simulink model "SimulArm_Sliders"  (R2025b)
settings: Solver=VariableStepAuto  StartTime=0.0  StopTime=100  RelTol=1e-3  AbsTol=1e-3  EnableMultiTasking=on
values from neighbouring files (symbols this model uses):
  C = U * V'    [DataCondition.m]
  g = 9.80665    [DataCondition.m]
  N = numel(raw)    [DataCondition.m]
undefined symbols (not defined in the file or in its folder): X, Y, Z
libraries: sm_lib x45, nesl_utility x24, aerolibconvert2 x5, simulink x1
(part 1 of 3)
settings Model: SimulationMode=accelerator  Creator=ricky  LastModifiedBy=ricky
settings SolverCC: AutoScaleAbsTol=off  AlgebraicLoopSolver=TrustRegion  MaxZcPerStep=1.0
settings DataIOCC: LimitDataPoints=on  MaxDataPoints=10000
settings OptimizationCC: ReuseModelBlockBuffer=off  LifeSpan=inf
settings DebuggingCC: UnconnectedInputMsg=warning  UnconnectedOutputMsg=warning  UnconnectedLineMsg=warning  AllowSymbolicDim=off  SubsystemReferenceDiagnosticForUnitTest=warning  SFUnexpectedBacktrackingDiag=warning  SFNoUnconditionalDefaultTransitionDiag=warning  SFExecutionAtInitializationDiag=none  ArithmeticOperatorsInVariantConditions=warning
settings ModelReferenceCC: EnableRefExpFcnMdlSchedulingChecks=on
settings SFSimCC: SimUseLocalCustomCode=off  CustomCodeUndefinedFunction=UseInterfaceOnly
settings RTWCC: RTWUseLocalCustomCode=off  GPUComputeCapability=3.5  DLArmComputeVersion=19.05
settings CodeAppCC: StateflowObjectComments=on
settings GRTTargetCC: TargetLangStandard=C89/C90 (ANSI)
settings ConfigComp: CovMetricSettings=dw  CovSaveCumulativeToWorkspaceVar=on  CovSaveSingleToWorkspaceVar=on  CovExternalEMLEnable=off  CovSFcnEnable=off
settings SimscapeCC: SimscapeLogType=all  SimscapeLogSimulationStatistics=on  SimscapeLogDataHistory=10000.0

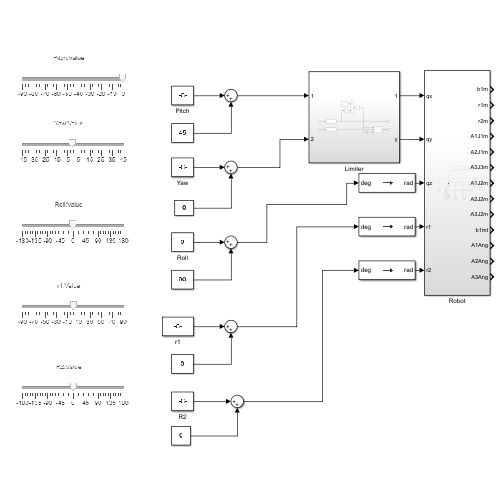
[thumbnail: Simulink's stored preview of the top-level diagram]
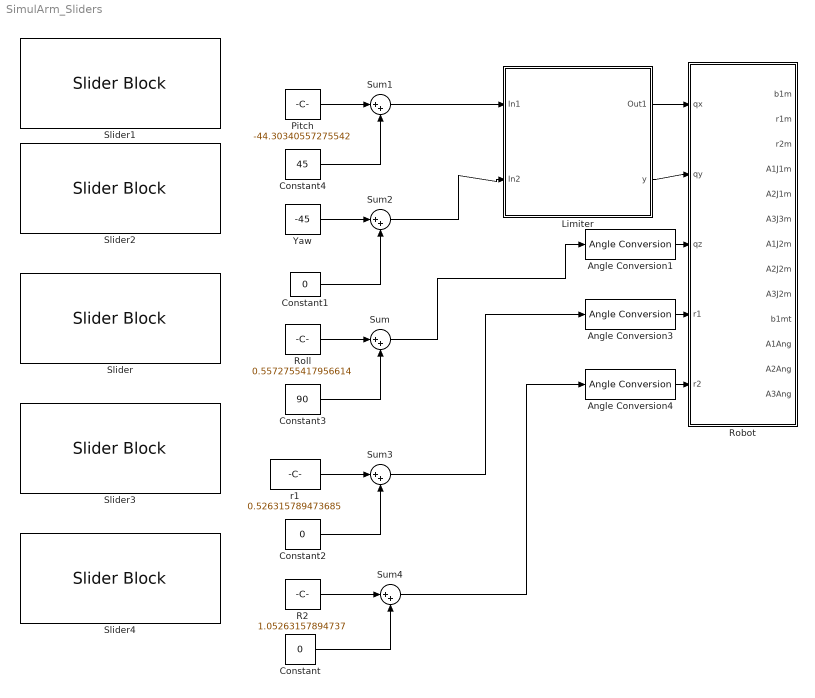
== system SimulArm_Sliders ==
  Angle Conversion1 : aerolibconvert2/Angle Conversion  IU=deg  OU=rad
  Angle Conversion3 : aerolibconvert2/Angle Conversion  IU=deg  OU=rad
  Angle Conversion4 : aerolibconvert2/Angle Conversion  IU=deg  OU=rad
  Constant : Constant  Value=0
  Constant1 : Constant  Value=0
  Constant2 : Constant  Value=0
  Constant3 : Constant  Value=90
  Constant4 : Constant  Value=45
  Limiter : Subsystem
  Pitch : Constant  Value=-44.30340557275542
  R2 : Constant  Value=1.05263157894737
  Robot : Subsystem
  Roll : Constant  Value=0.5572755417956614
  Slider : SliderBlock  ScaleMin=-180  ScaleMax=180
  Slider1 : SliderBlock  ScaleMin=-90  ScaleMax=0
  Slider2 : SliderBlock  ScaleMin=-45  ScaleMax=45
  Slider3 : SliderBlock  ScaleMin=-90  ScaleMax=90
  Slider4 : SliderBlock  ScaleMin=-180  ScaleMax=180
  Sum{,1..4} (5 alike) : Sum  Inputs=|++
  Yaw : Constant  Value=-45
  r1 : Constant  Value=0.526315789473685
  wires:
  Angle Conversion1/1 -> Robot/3(qz)
  Sum/1 -> Angle Conversion1/1
  Constant3/1 -> Sum/2
  Constant4/1 -> Sum1/2
  Constant1/1 -> Sum2/2
  Roll/1 -> Sum/1
  Angle Conversion3/1 -> Robot/4(r1)
  Angle Conversion4/1 -> Robot/5(r2)
  r1/1 -> Sum3/1
  Constant2/1 -> Sum3/2
  R2/1 -> Sum4/1
  Constant/1 -> Sum4/2
  Sum3/1 -> Angle Conversion3/1
  Sum4/1 -> Angle Conversion4/1
  Pitch/1 -> Sum1/1
  Yaw/1 -> Sum2/1
  Sum1/1 -> Limiter/1(In1)
  Sum2/1 -> Limiter/2(In2)
  Limiter/1(Out1) -> Robot/1(qx)
  Limiter/2(y) -> Robot/2(qy)

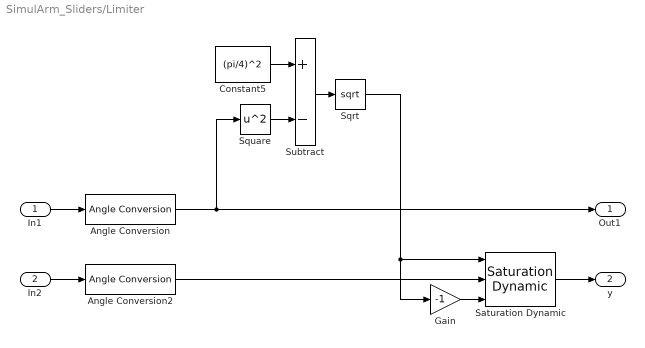
== system SimulArm_Sliders/Limiter ==
  In1 : Inport
  In2 : Inport  Port=2
  Angle Conversion : aerolibconvert2/Angle Conversion  IU=deg  OU=rad
  Angle Conversion2 : aerolibconvert2/Angle Conversion  IU=deg  OU=rad
  Constant5 : Constant  Value=(pi/4)^2
  Gain : Gain  Gain=-1
  Saturation Dynamic : simulink/Discontinuities/Saturation Dynamic  OutMin=[]  OutMax=[]  OutDataTypeStr=Inherit: Same as second input  OutDataType=fixdt(1, 16)  OutScaling=2^-10  DoSatur=off
  Sqrt : Sqrt
  Square : Math  Operator=square
  Subtract : Sum  Inputs=+-
  Out1 : Outport
  y : Outport  Port=2
  wires:
  Gain/1 -> Saturation Dynamic/3
  Angle Conversion2/1 -> Saturation Dynamic/2
  Sqrt/1 -> Gain/1, Saturation Dynamic/1
  Subtract/1 -> Sqrt/1
  Constant5/1 -> Subtract/1
  Angle Conversion/1 -> Out1/1, Square/1
  Square/1 -> Subtract/2
  In1/1 -> Angle Conversion/1
  Saturation Dynamic/1 -> y/1
  In2/1 -> Angle Conversion2/1
